simulink model "QpskSineMod"  (R2024a)
settings: Solver=VariableStepAuto  StartTime=0.0  StopTime=10.0  RelTol=1e-3
model workspace (MAT data in the model file):
  samp = 10
libraries: commdigbbndpm3 x1, commrandsrc3 x1
settings Model: Creator=Avinash  LastModifiedBy=Avinash

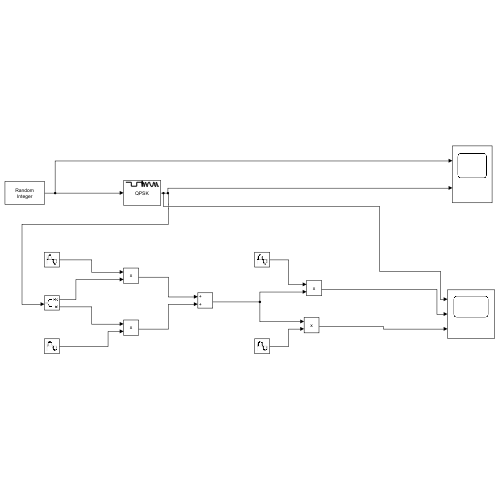
[thumbnail: Simulink's stored preview of the top-level diagram]
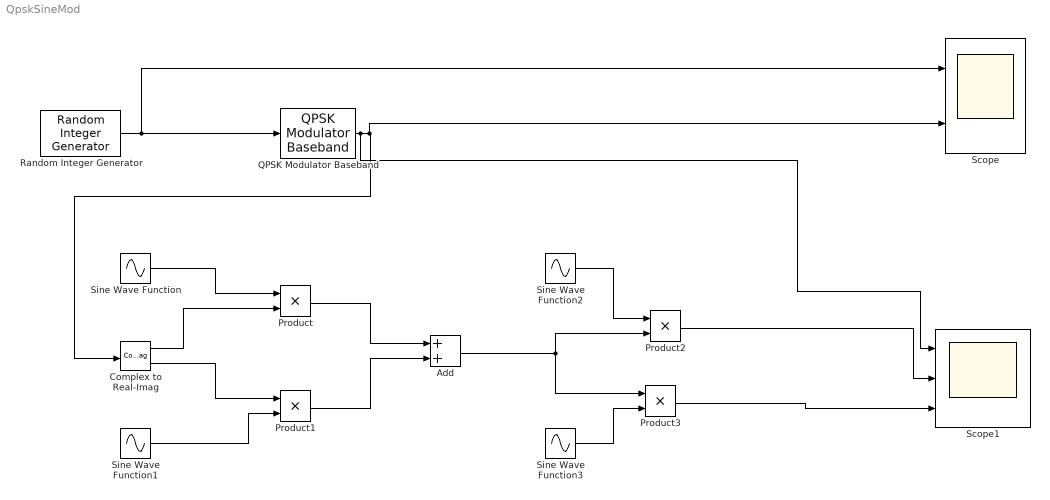
== system QpskSineMod ==
  Add : Sum
  Complex to Real-Imag : ComplexToRealImag
  Product{,1..3} (4 alike) : Product
  QPSK Modulator Baseband : commdigbbndpm3/QPSK Modulator Baseband  InType=Integer  Enc=Gray  Ph=pi/4  outDtype=double  outWordLen=16  outUDDataType=sfix(16)  outFracLenMode=Best precision  outFracLen=15  outDataTypeStr=double  outLastDataTypeStr=double
  Random Integer Generator : commrandsrc3/Random Integer Generator  SetSize=4  SeedSource=Auto  Seed=0  SampleTime=1  SamplesPerFrame=1  OutputDataType=double  SimulateUsing=Interpreted execution
  Scope : Scope  NumInputPorts=2
  Scope1 : Scope  NumInputPorts=3
  Sine Wave Function : Sin  Amplitude=samp  Frequency=4*2*pi  Phase=pi/2  SampleTime=0.001
  Sine Wave Function1 : Sin  Amplitude=samp  Frequency=4*2*pi  SampleTime=0.001
  Sine Wave Function2 : Sin  Amplitude=samp  Frequency=4*2*pi  Phase=pi/2  SampleTime=0.001
  Sine Wave Function3 : Sin  Amplitude=samp  Frequency=4*2*pi  SampleTime=0.001
  wires:
  Random Integer Generator/1 -> QPSK Modulator Baseband/1, Scope/1
  QPSK Modulator Baseband/1 -> Scope1/1, Scope/2, Complex to Real-Imag/1
  Sine Wave Function/1 -> Product/1
  Complex to Real-Imag/1 -> Product/2
  Complex to Real-Imag/2 -> Product1/1
  Sine Wave Function1/1 -> Product1/2
  Product1/1 -> Add/2
  Product/1 -> Add/1
  Add/1 -> Product3/1, Product2/2
  Sine Wave Function2/1 -> Product2/1
  Sine Wave Function3/1 -> Product3/2
  Product2/1 -> Scope1/2
  Product3/1 -> Scope1/3
